simulink model "Demo_V2XStats_Intersection_1_cs"  (R2014b)
settings: Solver=FixedStepDiscrete  SolverMode=SingleTasking  StartTime=0.0  StopTime=10  FixedStep=1/20  RelTol=1e-3
PreLoadFcn:
  | mbxruntime.callbacks.PreLoadFcn(bdroot);
  | check_NUTS_defined
  | model_closed = 0;
  | assignin('base',['model_closed_' bdroot],false);
PostLoadFcn:
  | mbxruntime.callbacks.PostLoadFcn(bdroot);
InitFcn:
  | mbxruntime.callbacks.InitFcn(bdroot);
StartFcn:
  | mbxruntime.callbacks.StartFcn(bdroot);
StopFcn:
  | mbxruntime.callbacks.StopFcn(bdroot);;
  | 
  | PostProcessing
  | 
model workspace: external: MAT-File .\Demo_V2XStats_Intersection_1_cs_hws.mat (data not in the file)
undefined symbols (not defined in the file or in its folder): InitializeBus, mbxruntime, tabledata
undefined symbols (not defined in the file): Demo_V2XStats_Intersection_1_cs_022fa72960d02a99, Demo_V2XStats_Intersection_1_cs_0667b7440011464a, Demo_V2XStats_Intersection_1_cs_0a717f3b1f82dce8, Demo_V2XStats_Intersection_1_cs_1912d0ac773e0614, Demo_V2XStats_Intersection_1_cs_1b4820430dd12493, Demo_V2XStats_Intersection_1_cs_3bba87328ee67e0a, Demo_V2XStats_Intersection_1_cs_467d7b57b3557fc2, Demo_V2XStats_Intersection_1_cs_534bad308c560994, Demo_V2XStats_Intersection_1_cs_58d6839509a0e403, Demo_V2XStats_Intersection_1_cs_7e2090151d7b4087, Demo_V2XStats_Intersection_1_cs_9888c4f7e8bf41a4, Demo_V2XStats_Intersection_1_cs_a103b1f27004d7b9, Demo_V2XStats_Intersection_1_cs_dde6e9b2bb85eae6, Demo_V2XStats_Intersection_1_cs_fcdd4688b7d5d124
libraries: simulink x5, PreScanSimulinkLibrary x4, PreScanUsefulBlocks x1, simulink_extras x1
(part 3 of 3)

== matlab function Demo_V2XStats_Intersection_1_cs/Nissan_Cabstar_1/V2X_2817_CAM_Create ==
  data: PRESCAN_V2X_FIXED_CAM_MESSAGE_zero_init parameter Bus: PRESCAN_V2X_FIXED_CAM_MESSAGE; message output Bus: PRESCAN_V2X_FIXED_CAM_MESSAGE; gpsLatLon input; altitude input; velocity input; longitudinalAcceleration input; heading input; yawRate input; generationDeltaTime input; vehicleLength input; vehicleWidth input; exteriorLights input
function message = update(PRESCAN_V2X_FIXED_CAM_MESSAGE_zero_init, gpsLatLon, altitude, velocity, longitudinalAcceleration, heading, yawRate, generationDeltaTime, vehicleLength, vehicleWidth, exteriorLights)
%#codegen

message = PRESCAN_V2X_FIXED_CAM_MESSAGE_zero_init;
message.HEADER.valid = true;

% The lines below are example assignments that can be uncommented
% and changed as needed to construct a message to be sent.

% message.DATA.header.protocolVersion = int32(1);
message.DATA.header.messageID = int32(2);
message.DATA.header.stationID = int32(4);
% message.DATA.cam.camParameters.basicContainer.referencePosition.positionConfidenceEllipse.semiMajorConfidence = int32(1);
% message.DATA.cam.camParameters.basicContainer.referencePosition.positionConfidenceEllipse.semiMinorConfidence = int32(1);
message.DATA.cam.camParameters.basicContainer.referencePosition.positionConfidenceEllipse.semiMajorOrientation = heading;
message.DATA.cam.camParameters.basicContainer.referencePosition.altitude.altitudeValue = altitude;
% message.DATA.cam.camParameters.basicContainer.referencePosition.altitude.altitudeConfidence = int32(1);
message.DATA.cam.camParameters.basicContainer.referencePosition.latitude = gpsLatLon(1);
message.DATA.cam.camParameters.basicContainer.referencePosition.longitude = gpsLatLon(2);
message.DATA.cam.camParameters.basicContainer.stationType = int32(5);
message.DATA.cam.camParameters.highFrequencyContainer.basicVehicleContainerHighFrequency.heading.headingValue = heading;
% message.DATA.cam.camParameters.highFrequencyContainer.basicVehicleContainerHighFrequency.heading.headingConfidence = int32(1);
message.DATA.cam.camParameters.highFrequencyContainer.basicVehicleContainerHighFrequency.speed.speedValue = velocity;
% message.DATA.cam.camParameters.highFrequencyContainer.basicVehicleContainerHighFrequency.speed.speedConfidence = int32(1);
message.DATA.cam.camParameters.highFrequencyContainer.basicVehicleContainerHighFrequency.vehicleLength.vehicleLengthValue = vehicleLength;
% message.DATA.cam.camParameters.highFrequencyContainer.basicVehicleContainerHighFrequency.vehicleLength.vehicleLengthConfidenceIndication = int32(1);
message.DATA.cam.camParameters.highFrequencyContainer.basicVehicleContainerHighFrequency.longitudinalAcceleration.longitudinalAccelerationValue = longitudinalAcceleration;
% message.DATA.cam.camParameters.highFrequencyContainer.basicVehicleContainerHighFrequency.longitudinalAcceleration.longitudinalAccelerationConfidence = int32(1);
% message.DATA.cam.camParameters.highFrequencyContainer.basicVehicleContainerHighFrequency.curvature.curvatureValue = int32(1);
% message.DATA.cam.camParameters.highFrequencyContainer.basicVehicleContainerHighFrequency.curvature.curvatureConfidence = int32(1);
message.DATA.cam.camParameters.highFrequencyContainer.basicVehicleContainerHighFrequency.yawRate.yawRateValue = yawRate;
% message.DATA.cam.camParameters.highFrequencyContainer.basicVehicleContainerHighFrequency.yawRate.yawRateConfidence = int32(1);
% message.DATA.cam.camParameters.highFrequencyContainer.basicVehicleContainerHighFrequency.steeringWheelAngle.steeringWheelAngleValue = int32(1);
% message.DATA.cam.camParameters.highFrequencyContainer.basicVehicleContainerHighFrequency.steeringWheelAngle.steeringWheelAngleConfidence = int32(1);
% message.DATA.cam.camParameters.highFrequencyContainer.basicVehicleContainerHighFrequency.lateralAcceleration.lateralAccelerationValue = int32(1);
% message.DATA.cam.camParameters.highFrequencyContainer.basicVehicleContainerHighFrequency.lateralAcceleration.lateralAccelerationConfidence = int32(1);
% message.DATA.cam.camParameters.highFrequencyContainer.basicVehicleContainerHighFrequency.verticalAcceleration.verticalAccelerationValue = int32(1);
% message.DATA.cam.camParameters.highFrequencyContainer.basicVehicleContainerHighFrequency.verticalAcceleration.verticalAccelerationConfidence = int32(1);
% message.DATA.cam.camParameters.highFrequencyContainer.basicVehicleContainerHighFrequency.cenDsrcTollingZone.protectedZoneLatitude = int32(1);
% message.DATA.cam.camParameters.highFrequencyContainer.basicVehicleContainerHighFrequency.cenDsrcTollingZone.protectedZoneLongitude = int32(1);
% message.DATA.cam.camParameters.highFrequencyContainer.basicVehicleContainerHighFrequency.cenDsrcTollingZone.cenDsrcTollingZoneID = int32(1);
% message.DATA.cam.camParameters.highFrequencyContainer.basicVehicleContainerHighFrequency.driveDirection = int32(1);
message.DATA.cam.camParameters.highFrequencyContainer.basicVehicleContainerHighFrequency.vehicleWidth = vehicleWidth;
% message.DATA.cam.camParameters.highFrequencyContainer.basicVehicleContainerHighFrequency.curvatureCalculationMode = int32(1);
% message.DATA.cam.camParameters.highFrequencyContainer.basicVehicleContainerHighFrequency.accelerationControl = int32(1);
% message.DATA.cam.camParameters.highFrequencyContainer.basicVehicleContainerHighFrequency.lanePosition = int32(1);
% message.DATA.cam.camParameters.highFrequencyContainer.basicVehicleContainerHighFrequency.performanceClass = int32(1);
% message.DATA.cam.camParameters.highFrequencyContainer.rsuContainerHighFrequency.protectedCommunicationZonesRSU(1).protectedZoneType = int32(1);
% message.DATA.cam.camParameters.highFrequencyContainer.rsuContainerHighFrequency.protectedCommunicationZonesRSU(1).expiryTime = int32(1);
% message.DATA.cam.camParameters.highFrequencyContainer.rsuContainerHighFrequency.protectedCommunicationZonesRSU(1).protectedZoneLatitude = int32(1);
% message.DATA.cam.camParameters.highFrequencyContainer.rsuContainerHighFrequency.protectedCommunicationZonesRSU(1).protectedZoneLongitude = int32(1);
% message.DATA.cam.camParameters.highFrequencyContainer.rsuContainerHighFrequency.protectedCommunicationZonesRSU(1).protectedZoneRadius = int32(1);
% message.DATA.cam.camParameters.highFrequencyContainer.rsuContainerHighFrequency.protectedCommunicationZonesRSU(1).protectedZoneID = int32(1);
% % message.DATA.cam.camParameters.highFrequencyContainer.rsuContainerHighFrequency.protectedCommunicationZonesRSU(1) is an array
% message.DATA.cam.camParameters.lowFrequencyContainer.basicVehicleContainerLowFrequency.pathHistory(1).pathPosition.deltaLatitude = int32(1);
% message.DATA.cam.camParameters.lowFrequencyContainer.basicVehicleContainerLowFrequency.pathHistory(1).pathPosition.deltaLongitude = int32(1);
% message.DATA.cam.camParameters.lowFrequencyContainer.basicVehicleContainerLowFrequency.pathHistory(1).pathPosition.deltaAltitude = int32(1);
% message.DATA.cam.camParameters.lowFrequencyContainer.basicVehicleContainerLowFrequency.pathHistory(1).pathDeltaTime = int32(1);
% message.DATA.cam.camParameters.lowFrequencyContainer.basicVehicleContainerLowFrequency.vehicleRole = int32(1);
message.DATA.cam.camParameters.lowFrequencyContainer.basicVehicleContainerLowFrequency.exteriorLights = exteriorLights;
% % message.DATA.cam.camParameters.lowFrequencyContainer.basicVehicleContainerLowFrequency.pathHistory(1) is an array
% message.DATA.cam.camParameters.specialVehicleContainer.publicTransportContainer.ptActivation.ptActivationType = int32(1);
% message.DATA.cam.camParameters.specialVehicleContainer.publicTransportContainer.ptActivation.ptActivationData = int8(zeros(20, 1)); % Array up to 20 bytes
% message.DATA.cam.camParameters.specialVehicleContainer.publicTransportContainer.embarkationStatus = logical(1);
% message.DATA.cam.camParameters.specialVehicleContainer.specialTransportContainer.specialTransportType = int32(1);
% message.DATA.cam.camParameters.specialVehicleContainer.specialTransportContainer.lightBarSirenInUse = int32(1);
% message.DATA.cam.camParameters.specialVehicleContainer.dangerousGoodsContainer.dangerousGoodsBasic = int32(1);
% message.DATA.cam.camParameters.specialVehicleContainer.roadWorksContainerBasic.closedLanes.hardShoulderStatus = int32(1);
% message.DATA.cam.camParameters.specialVehicleContainer.roadWorksContainerBasic.closedLanes.drivingLaneStatus = int32(1);
% message.DATA.cam.camParameters.specialVehicleContainer.roadWorksContainerBasic.roadworksSubCauseCode = int32(1);
% message.DATA.cam.camParameters.specialVehicleContainer.roadWorksContainerBasic.lightBarSirenInUse = int32(1);
% message.DATA.cam.camParameters.specialVehicleContainer.rescueContainer.lightBarSirenInUse = int32(1);
% message.DATA.cam.camParameters.specialVehicleContainer.emergencyContainer.incidentIndication.causeCode = int32(1);
% message.DATA.cam.camParameters.specialVehicleContainer.emergencyContainer.incidentIndication.subCauseCode = int32(1);
% message.DATA.cam.camParameters.specialVehicleContainer.emergencyContainer.lightBarSirenInUse = int32(1);
% message.DATA.cam.camParameters.specialVehicleContainer.emergencyContainer.emergencyPriority = int32(1);
% message.DATA.cam.camParameters.specialVehicleContainer.safetyCarContainer.incidentIndication.causeCode = int32(1);
% message.DATA.cam.camParameters.specialVehicleContainer.safetyCarContainer.incidentIndication.subCauseCode = int32(1);
% message.DATA.cam.camParameters.specialVehicleContainer.safetyCarContainer.lightBarSirenInUse = int32(1);
% message.DATA.cam.camParameters.specialVehicleContainer.safetyCarContainer.trafficRule = int32(1);
% message.DATA.cam.camParameters.specialVehicleContainer.safetyCarContainer.speedLimit = int32(1);
message.DATA.cam.generationDeltaTime = generationDeltaTime;
